simulink model "Saved_model"  (R2018b)
settings: Solver=VariableStepAuto  StartTime=0.0  StopTime=10.0  RelTol=1e-3
settings Model: Creator=LaAir  LastModifiedBy=LaAir

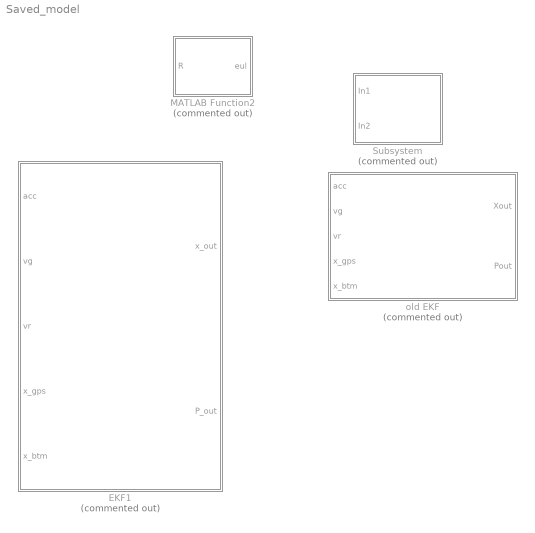
== system Saved_model ==
  EKF1 : MATLAB Function  Commented=on  TreatAsAtomicUnit=on  SystemSampleTime=1e-3
  MATLAB Function2 : MATLAB Function  Commented=on  TreatAsAtomicUnit=on
  Subsystem : Subsystem  Commented=on
  old EKF : MATLAB Function  Commented=on  TreatAsAtomicUnit=on  SystemSampleTime=1e-3

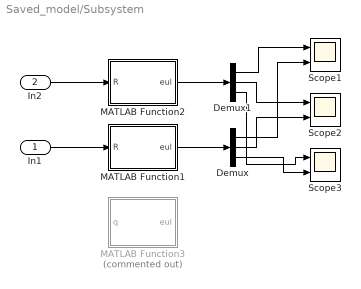
== system Saved_model/Subsystem ==
  In1 : Inport
  In2 : Inport  Port=2
  Demux : Demux  Outputs=3
  Demux1 : Demux  Outputs=3
  MATLAB Function1 : MATLAB Function  TreatAsAtomicUnit=on
  MATLAB Function2 : MATLAB Function  TreatAsAtomicUnit=on
  MATLAB Function3 : MATLAB Function  Commented=on  TreatAsAtomicUnit=on
  Scope1 : Scope  NumInputPorts=2
  Scope2 : Scope  NumInputPorts=2
  Scope3 : Scope  NumInputPorts=2
  wires:
  Demux/1 -> Scope1/2
  Demux/3 -> Scope3/2
  MATLAB Function1/1(eul) -> Demux/1
  In2/1 -> MATLAB Function2/1(R)
  MATLAB Function2/1(eul) -> Demux1/1
  Demux1/1 -> Scope1/1
  Demux1/3 -> Scope3/1
  Demux1/2 -> Scope2/1
  Demux/2 -> Scope2/2
  In1/1 -> MATLAB Function1/1(R)

== matlab function Saved_model/EKF1 ==
  data: acc input; x_out output; vg input; vr input; x_gps input; x_btm input; P_out output
function [x_out, P_out] = fcn(acc, vg, vr, x_gps, x_btm)
% 状态: x=[ x; v; b_a; s_w ], 位置/速度/加速度零偏/轮速尺度(≈1+ε)
% 缺测用 NaN；兼容旧工程，位置=0/速度=0 也可视为缺测，但做了低速保护避免误杀真零速

dt = 1e-3;

persistent x P inited
if isempty(inited)
    x = [0; 0; 0; 1.0];
    P = diag([100, 10, 0.1, 1e-2]);
    inited = true;
end

% ---------- 观测缺测兼容层 ----------
% 优先 isnan；保留兼容
if nargin < 5, x_btm = NaN; end
if nargin < 4, x_gps = NaN; end

if ~isnan(x_gps) && x_gps==0, x_gps = NaN; end
if ~isnan(x_btm) && x_btm==0, x_btm = NaN; end

% 速度类：0 既可能是真零速也可能是缺测；若当前状态 |v| 明显非零，则把 0 当缺测
v_now = x(2);
if ~isnan(vg) && vg==0 && abs(v_now)>0.2, vg = NaN; end
if ~isnan(vr) && vr==0 && abs(v_now)>0.2, vr = NaN; end

% 加速度预处理
acc_t = acc(1);
if any(isnan(acc_t)), acc_t = 0; end
a = acc_t;   % 已在外部完成姿态投影到轨道切向

% ---------- 过程模型 ----------
% x = [x; v; b_a; s_w]
F = eye(4);
F(1,2) = dt;     % dx/dv
F(2,3) = -dt;    % dv/db_a

% 过程噪声（经验值，可再调）
sigma_a  = 0.6;          % m/s^2  加计噪声等效
sigma_b  = 1e-3;         % (m/s^2)/sqrt(s)  加计零偏随机游走
sigma_sw = 1e-5;         % 轮径尺度随机游走 /sqrt(s)
G = [0.5*dt^2; dt; 0; 0];  % 加速度噪声驱动到 [x;v]
Q = zeros(4);
Q = Q + (sigma_a^2)*(G*G.');
Q(3,3) = Q(3,3) + (sigma_b^2)*dt;
Q(4,4) = Q(4,4) + (sigma_sw^2)*dt;

% 预测
x = [ x(1) + x(2)*dt;
      x(2) + (a - x(3))*dt;
      x(3);
      x(4) ];
P = F*P*F' + Q;

% 保证 s_w 正且不过分跑飞（简单夹紧）
x(4) = max(0.7, min(1.3, x(4)));

% ---------- 观测与更新 ----------
% h(x):
%   GPS:   x
%   BTM:   x
%   轮速:  s_w * v
%   雷达:  v
H_full = [ 1 0 0 0;          % GPS
           1 0 0 0;          % BTM
           0 x(4) 0 x(2);    % 轮速的正确雅可比！！
           0 1   0 0  ];     % 雷达

z_full = [x_gps; x_btm; vg; vr];

% 测量噪声
sigma_gps = 2.0;    % m
sigma_btm = 0.5;    % m
sigma_vr  = 0.25;   % m/s
% 轮速噪声：基线 + 随速度变化；低速时观测对 s_w 不可观/容易滑差，抬高噪声或跳过
v_abs = abs(x(2));
sigma_vg = 0.05 + 5e-3*v_abs;  % m/s
R_full = diag([sigma_gps^2, sigma_btm^2, sigma_vg^2, sigma_vr^2]);

% 低速保护与防滑（关键）：
% 1) |v| 很小 → 不更新轮速项（对 s_w 几乎不可观）
% 2) 残差过大 → 判定打滑，仅临时放大轮速 R，而不是整条观测抛弃
mask = ~isnan(z_full);
if v_abs < 0.2           % 低速阈值，可调
    mask(3) = false;     % 暂不使用轮速
end

if any(mask)
    H = H_full(mask, :);
    z = z_full(mask);
    R = R_full(mask, mask);

    % 非线性观测值
    h = zeros(nnz(mask),1);
    idx = find(mask);
    for k = 1:numel(idx)
        switch idx(k)
            case 1, h(k) = x(1);           % GPS
            case 2, h(k) = x(1);           % BTM
            case 3, h(k) = x(4)*x(2);      % 轮速
            case 4, h(k) = x(2);           % 雷达
        end
    end

    % 残差预计算
    r = z - h;

    % 若包含轮速项，做一次“打滑检测”：|r_vg| > 3σ → 放大该项 R（例如 ×25）
    if any(idx==3)
        pos = find(idx==3,1,'first');           % 轮速在子观测向量的位置
        if abs(r(pos)) > 3*sqrt(R(pos,pos))
            R(pos,pos) = 25*R(pos,pos);         % 软抑制轮速而非丢弃
        end
    end

    % 标准 EKF 更新
    S = H*P*H' + R;
    K = P*H'/S;
    x = x + K*(z - h);
    P = (eye(4) - K*H)*P*(eye(4) - K*H)' + K*R*K';
end

x_out = x;
P_out = P;
end

== matlab function Saved_model/MATLAB Function2 ==
  data: R input; eul output
 function eul = deg(R)
[U, ~, V] = svd(R);
R = U * V';
yaw = atan2(R(2,1),R(1,1));
pitch = asin(-R(3,1));
roll = atan2(R(3,2),R(3,3));
eul = [yaw, pitch, roll]*180/pi;

== matlab function Saved_model/Subsystem/MATLAB Function1 ==
  data: R input; eul output
 function eul = rad(R)
[U, ~, V] = svd(R);
R = U * V';
yaw = atan2(R(2,1),R(1,1));
pitch = asin(-R(3,1));
roll = atan2(R(3,2),R(3,3));
eul = [yaw, pitch, roll];

== matlab function Saved_model/Subsystem/MATLAB Function2 ==
  data: R input; eul output
 function eul = rad(R)
[U, ~, V] = svd(R);
R = U * V';
yaw = atan2(R(2,1),R(1,1));
pitch = asin(-R(3,1));
roll = atan2(R(3,2),R(3,3));
eul = [yaw, pitch, roll];

== matlab function Saved_model/Subsystem/MATLAB Function3 ==
  data: q input; eul output
function eul = q2eul(q)
% 输入 q = [qw qx qy qz]，Hamilton 定义（qw 是实部）
% 输出 yaw(Z)、pitch(Y)、roll(X)，单位 rad

    % 拆分
    qw = q(1); qx = q(2); qy = q(3); qz = q(4);

    % 旋转矩阵
    R = [ 1 - 2*(qy^2 + qz^2),   2*(qx*qy - qz*qw),   2*(qx*qz + qy*qw);
          2*(qx*qy + qz*qw),     1 - 2*(qx^2 + qz^2), 2*(qy*qz - qx*qw);
          2*(qx*qz - qy*qw),     2*(qy*qz + qx*qw),   1 - 2*(qx^2 + qy^2) ];

    % ZYX 欧拉角
    yaw   = atan2(R(2,1), R(1,1));      % ψ (Z)
    pitch = asin(-R(3,1));              % θ (Y)
    roll  = atan2(R(3,2), R(3,3));      % φ (X)
    eul = [yaw, pitch, roll];
end

== matlab function Saved_model/old EKF ==
  data: acc input; Xout output; vg input; vr input; x_gps input; x_btm input; Pout output
function [Xout, Pout] = fcn(acc, vg, vr, x_gps, x_btm)
dt = 1e-3;
if isnan(acc)
    acc = [0;0;0];
end

% 状态空间为: xs vs vx vy vz vgb
% vgb为轮径补偿
persistent X0 X1 P0 P1;
if isempty(X0)
    X0 = [0;0;0;0;0;0];
    X1 = [0;0;0;0;0;0];
    P0 = diag([100, 10, 10, 10, 10, 1]);
    P1 = diag([100, 10, 10, 10, 10, 1]);
end

% 协方差
Ra = diag([0,0,0.5,0.5,0.5,0]);
Q = eye(6)*0.1;
Z_org = [x_gps; x_btm; vg; vr];
P_m_org = diag([10^2, 0.1^2, 0.1^2, (0.3+X0(2)*5e-3)^2]);


% select
has_vg = (vg ~= 0);
has_vr = (vr ~= 0);
has_gps = (x_gps ~= 0);
has_btm = ( x_btm ~= 0);
mask = [has_gps, has_btm, has_vg, has_vr];
H_org = [1 0 0 0 0 0;
        1 0 0 0 0 0;
        0 1 0 0 0 1;
        0 1 0 0 0 1];
H = H_org(mask,:);
P_m = P_m_org(mask,mask);
Z = Z_org(mask);

% update
if ~isempty(H)
    K = P0*H' * (H*P0*H' + P_m)^-1;
    P1 = (eye(6)-K*H)*P0;
    X1 = X0 + K*(Z-H*X0);
else
    X1 = X0;
    P1 = P0;
end

% predict
X0(1) = X1(1) + X1(2)*dt;
X0(2) = norm(X1(2:4));
X0(3) = X1(3) + acc(1)*dt;
X0(4) = X1(4) + acc(2)*dt;
X0(5) = X1(5) + acc(3)*dt;
X0(6) = X1(6);

F = [1 dt 0 0 0 0;
    0 1 X1(3)/X1(2) X1(4)/X1(2) X1(5)/X1(2) 0;
    0 0 1 0 0 0;
    0 0 0 1 0 0;
    0 0 0 0 1 0;
    0 0 0 0 0 1];
P0 = F*P1*F' + Ra + Q*dt^2;
Xout = X0;
Pout = P0;
